simulink model "Model_1_Simple_Linear_System"  (R2025b)
settings: Solver=ode1  StartTime=0.0  StopTime=10.0  FixedStep=0.4  MaxStep=0.5  MinStep=0.1  RelTol=1e-3
settings Model: Creator=danielborkovec  LastModifiedBy=danielborkovec
settings SolverCC: InitialStep=0.1
settings DataIOCC: SaveFormat=Array  ReturnWorkspaceOutputs=off

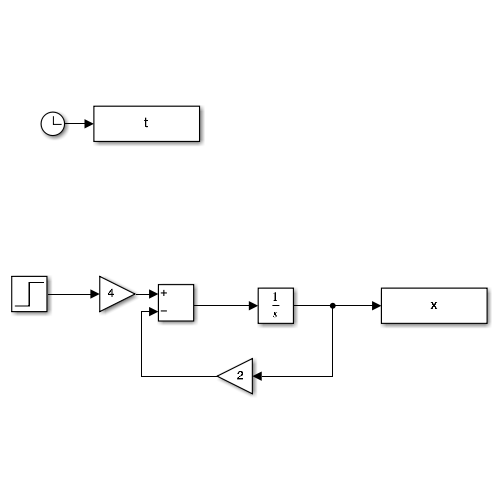
[thumbnail: Simulink's stored preview of the top-level diagram]
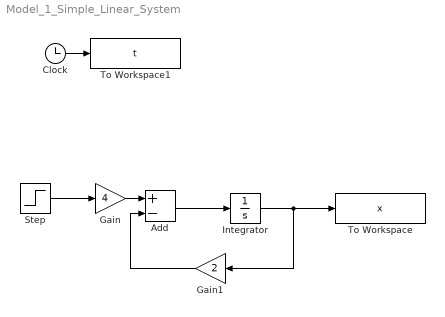
== system Model_1_Simple_Linear_System ==
  Add : Sum  Inputs=+-
  Clock : Clock
  Gain : Gain  Gain=4
  Gain1 : Gain  Gain=2
  Integrator : Integrator
  Step : Step  SampleTime=0
  To Workspace : ToWorkspace  VariableName=x  SampleTime=-1
  To Workspace1 : ToWorkspace  VariableName=t  SampleTime=-1
  wires:
  Clock/1 -> To Workspace1/1
  Step/1 -> Gain/1
  Gain/1 -> Add/1
  Add/1 -> Integrator/1
  Integrator/1 -> Gain1/1, To Workspace/1
  Gain1/1 -> Add/2
